simulink model "datatypes"  (R2017a)
settings: Solver=VariableStepAuto  StartTime=0.0  StopTime=10.0  RelTol=1e-3
settings Model: Creator=ptracton  LastModifiedBy=ptracton

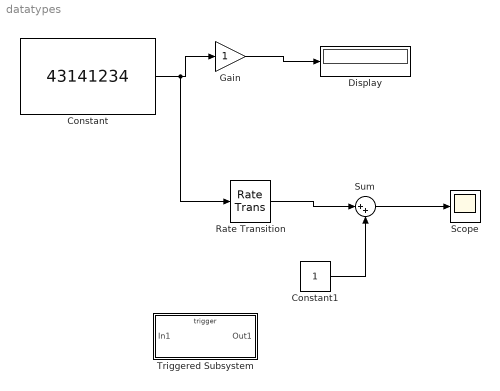
== system datatypes ==
  Constant : Constant  Value=43141234  OutDataTypeStr=boolean
  Constant1 : Constant  SampleTime=0.010
  Display : Display
  Gain : Gain  OutDataTypeStr=Inherit: Same as input
  Rate Transition : RateTransition
  Scope : Scope
  Sum : Sum  Inputs=|++
  Triggered Subsystem : Subsystem  TreatAsAtomicUnit=on
  wires:
  Constant/1 -> Rate Transition/1, Gain/1
  Gain/1 -> Display/1
  Constant1/1 -> Sum/2
  Rate Transition/1 -> Sum/1
  Sum/1 -> Scope/1

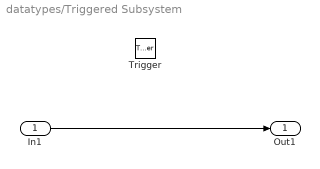
== system datatypes/Triggered Subsystem ==
  In1 : Inport
  Trigger : TriggerPort  VariantControl=Variant
  Out1 : Outport
  wires:
  In1/1 -> Out1/1
